simulink model "ADCCalibrationCAN"  (R2026a)
settings: Solver=FixedStepAuto  StopTime=inf  FixedStep=Ts_CPU  EnableMultiTasking=on
InitFcn:
  | Ts = 1e-4;
  | Tcpu = 50e-6; %Controller sample time
  | 
  | % PMSM parameters
  | PM = 0.03; % Permanent magnet flux linkage
  | Ld = 2e-4;  % d-axis inductance
  | Lq = 2e-4;  % q-axis inductance
  | L0 = 2e-4;  % 0-axis inductance
  | Rs = 0.013; % Stator resistance
  | N = 6; % Number of pole pairs
  | J = 0.2; % Moment of inertia
  | 
  | % encoder parameters
  | numSlits = 2000; % number of slits
  | pulseSigOffset = 0; % index pulse signal offset
  | shaftInitPos = 0; % motor shaft initial position
  | 
  | % DAC parameters
  | gain = 0.1;
  | bias = 0;
  | 
  | % circuit parameters
  | Vdc = 48;
  | 
  | % real-time parameters
  | ts_FPGA_clk = 5e-9;
  | ts_FPGA_mdl = 1e-6;
  | 
  | % Real-time processor or embedded controller
  | RTorTTL = 1; % 1: Real-time processor,    0: embedded controller
  | 
  | % sample times
  | f_base = 200e6;
  | PWM_frequency = 20e3;
  | ts_FPGA_clk = 1/f_base;
  | ts_FPGA_mdl =1e-6;
undefined symbols (not defined in the file or in its folder): Foc_Ki_IxTcpu, Foc_Kp_I, IO334, IO334_iDAC_bias, IO334_iDAC_gain, Maxon_645604_J, Maxon_645604_lambda_pm, Maxon_645604_Ld, Maxon_645604_Lq, Maxon_645604_Np, Maxon_645604_Rs, Maxon_645604_StaticF, Maxon_645604_ViscousF, PMSM3P2LInverter_limited, PMSM_3P2L_Inverter_Plant, Ts_CAN_Tx, Ts_CPU, Ts_UI
libraries: speedgoatlib_hdlCoder_IO3xx x31, canmsglib x7, speedgoatlib_IO611 x3, pwm_cpulib x1, quadrature_cpulib x1, resolver_cpulib x1
(part 1 of 2)
settings Model: DataDictionary=PMSM3P2LInverterDd.sldd  EnableAccessToBaseWorkspace=off  SimulationMode=external  ExtModeEnableFloating=off  Creator=chrisz  LastModifiedBy=mathieu.lu-dac
settings SolverCC: ConcurrentTasks=on  PositivePriorityOrder=on
settings OptimizationCC: ConditionallyExecuteInputs=off  OptimizeBlockIOStorage=off
settings DebuggingCC: AlgebraicLoopMsg=error  SingleTaskRateTransMsg=error  TasksWithSamePriorityMsg=none  ParameterOverflowMsg=warning  ParameterUnderflowMsg=warning
settings HardwareCC: ProdBitPerLong=64.0  ProdHWDeviceType=Intel->x86-64 (Linux 64)  TargetBitPerPointer=64.0  TargetBitPerSizeT=64.0  TargetBitPerPtrDiffT=64.0  TargetLongLongMode=on  TargetIntDivRoundTo=Zero  TargetEndianess=LittleEndian  TargetWordSize=64.0  TargetHWDeviceType=Custom Processor->MATLAB Host Computer
settings RTWCC: SystemTargetFile=speedgoat.tlc  TemplateMakefile=slrealtime_default_tmf  Toolchain=Simulink Real-Time Toolchain  BuildConfiguration=Faster Runs  TargetLang=C++  Description=Speedgoat Real-Time Target Machine
settings SimulinkRealTimeTargetCC: SLRTFileLogMaxRuns=1.0  MultiwordLength=2048.0
settings SimscapeCC: SimscapeNominalValues="[{\"value\":\"1\",\"unit\":\"A\"},{\"value\":\"1\",\"unit\":\"bar\"},{\"value\":\"1\",\"unit\":\"cm^2\"},{\"value\":\"1\",\"unit\":\"cm^3/s\"},{\"value\":\"1\",\"unit\":\"kJ/kg\"},{\"value\":\"1\",\"unit\":\"kW\"},{\"value\":\"1\",\"unit\":\"l\"},{\"value\":\"1\",\"unit\":\"N\"},{\"value\":\"1\",\"unit\":\"N*m\"},{\"value\":\"1\",\"unit\":\"V\"}]"  SimscapeLogType=none  SimscapeLogDataHistory=5000.0

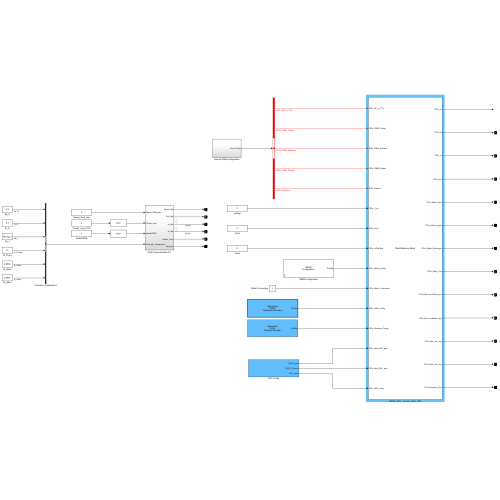
[thumbnail: Simulink's stored preview of the top-level diagram]
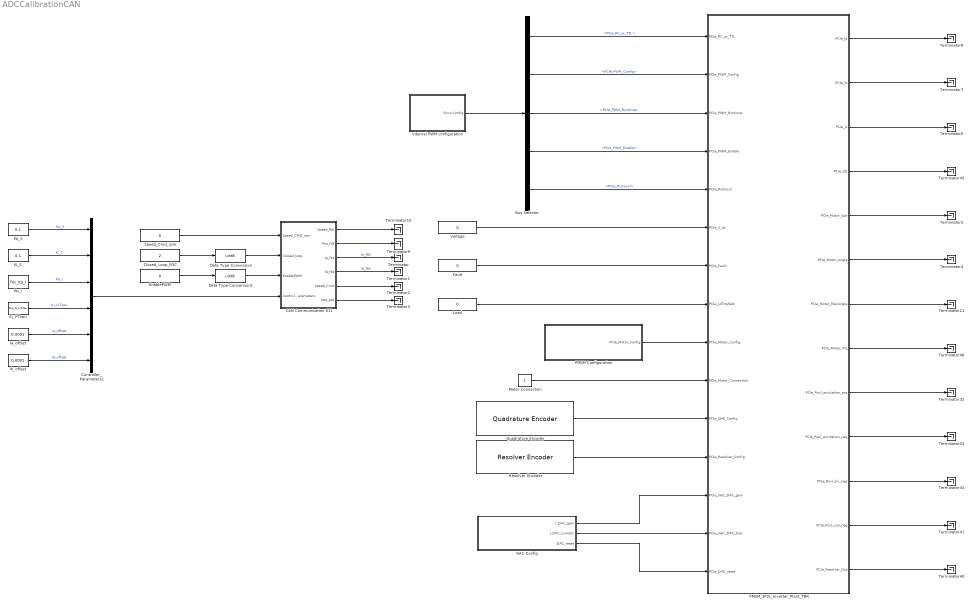
== system ADCCalibrationCAN ==
  Bus Selector : BusSelector  OutputSignals=PCIe_RC_or_TTL,PCIe_PWM_Config,PCIe_PWM_Runtime,PCIe_PWM_Enable,PCIe_Protocol
  CAN Communication 611 : Subsystem
  Closed_Loop_FOC : Constant  Value=2  OutDataTypeStr=uint8  SampleTime=Ts_UI
  Controller_Parameters1 : BusCreator  Inputs=6
  DAC Config : Subsystem
  Data Type Conversion : DataTypeConversion  OutDataTypeStr=uint8  SaturateOnIntegerOverflow=off  RndMeth=Floor
  Data Type Conversion1 : DataTypeConversion  OutDataTypeStr=uint8  SaturateOnIntegerOverflow=off  RndMeth=Floor
  EnablePWM : Constant  Value=0  OutDataTypeStr=boolean  SampleTime=Ts_UI
  Fault : Constant  Value=0  OutDataTypeStr=uint32  SampleTime=Ts_UI
  Ia_offset : Constant  Value=0.0001  OutDataTypeStr=single  SampleTime=Ts_UI
  Ib_offset : Constant  Value=0.0001  OutDataTypeStr=single  SampleTime=Ts_UI
  Internal PWM configuration : Subsystem
  Ki_S : Constant  Value=0.1  OutDataTypeStr=single  SampleTime=Ts_UI
  Ki_i*Tcpu : Constant  Value=Foc_Ki_IxTcpu  OutDataTypeStr=single  SampleTime=Ts_UI
  Kp_I : Constant  Value=Foc_Kp_I  OutDataTypeStr=single  SampleTime=Ts_UI
  Kp_S : Constant  Value=0.1  OutDataTypeStr=single  SampleTime=Ts_UI
  Load : Constant  Value=0  OutDataTypeStr=single  SampleTime=Ts_UI
  Motor Connection : Constant  OutDataTypeStr=boolean
  PMSM Configuration : Subsystem  InitFcn=|  mask(PMSM Configuration){portConfig=Torque, Trq_N_mode=0, Ts=Ts_CPU, Pp=Maxon_645604_Np, Rs=Maxon_645604_Rs, Ld=Maxon_645604_Ld, Lq=Maxon_645604_Lq, lambda_pm=Maxon_645604_lambda_pm, J=Maxon_645604_J, B=Maxon_645604_ViscousF*100, f=Maxon_645604_StaticF}
      | mcb.internal.manageMCBResource('register',gcbh);
      | mcb.internal.logDDUXData;
      mask prompts: portConfig "mcb:PlantLib:CfgMechInCfg"; Ts "mcb:PlantLib:CfgTs"; Pp "mcb:PlantLib:PMSMCfgPp"; Rs "mcb:PlantLib:PMSMCfgRs"; Ld "mcb:PlantLib:PMSMCfgLd"; Lq "mcb:PlantLib:PMSMCfgLq"; lambda_pm "mcb:PlantLib:PMSMCfgLambda"; J "mcb:PlantLib:PMSMCfgJ"; B "mcb:PlantLib:PMSMCfgB"; f "mcb:PlantLib:PMSMCfgf"
      mask help: mcb:PlantLib:PMSMCfgDes
      mask Help: eval('mcb_helpview(''pmsmhdlconfig'')')
      mask TypeOptions portConfig: mcb:PlantLib:CfgTorque | mcb:PlantLib:CfgSpd
      mask Callback portConfig:
      | %Do not run initialization code if model is running
      | invalidStatus = {'external','running','compiled','restarting','paused','terminating'};
      | if ~any(strcmpi(get_param(bdroot(gcb),'SimulationStatus'),invalidStatus))
      |     % Check the value selected in the pop-up
      |     mask = Simulink.Mask.get(gcb);
      |     portConfigStr = get_param(gcb, 'portConfig');
      |     if strcmp(portConfigStr, 'Torque')
      |         % Set Trq_N_mode value to 0
      |         mask.getParameter('Trq_N_mode').Value = '0';
      | 
      |     elseif strcmp(portConfigStr, 'Speed')
      |         % Set Trq_N_mode value to 2
      |         mask.getParameter('Trq_N_mode').Value = '1';
      | 
      |     end
      | end
      mask DialogControl DescGroupVar Prompt: mcb:PlantLib:PMSMCfgTitle
      mask DialogControl ParameterGroupVar Prompt: mcb:PlantLib:CfgBlk
      mask DialogControl portConfig Prompt: Mechanical input configuration:
      mask DialogControl Ts Prompt: Sample time (s):
      mask DialogControl Container4 Prompt: mcb:PlantLib:CfgParam
      mask DialogControl Pp Prompt: Number of pole pairs:
      mask DialogControl Rs Prompt: Stator resistance per phase (Ohm):
      mask DialogControl Ld Prompt: Stator d-axis inductance (H):
      mask DialogControl Lq Prompt: Stator q-axis inductance (H):
      mask DialogControl lambda_pm Prompt: Permanent flux linkage constant (Wb):
      mask DialogControl J Prompt: Inertia (kgm^2):
      mask DialogControl B Prompt: Viscous damping (Nm/rad/s):
      mask DialogControl f Prompt: Static friction (Nm):
      mask Display:
      | disp('PMSM\nConfiguration');
      | port_label('output',1,'Config');
  PMSM_3P2L_Inverter_Plant_TBR : Subsystem
      mask Display: disp('Plant Bitstream Block')
  Quadrature Encoder : quadrature_cpulib/Quadrature Encoder  FPGA_freq=f_FPGA  n_channels=[1]  sel_scaling=FPGA  useSpeed=off  usePosition=on  numOfSlots=Maxon_Mile_Nslits  sigAswitchOn=[180]  sigBswitchOff=[90]  sigBswitchOn=[270]  sigAdismissEn=off  sigAdismissSingle=on  sigAdismissHigh=on  sigBdismissEn=off  sigBdismissSingle=on  sigBdismissHigh=on
      settings: SourceProductName=Quadrature CPU Library
  Resolver Encoder : resolver_cpulib/Resolver Encoder  Ts=Ts_UI  ts_resolver=ts_FPGA_mdl  n_channels=1  sel_scaling=FPGA  useSpeed=on  usePosition=off  pole_pairs=1  gain_dynamic=off  gainVector=[1, 1, 1, 1]  offset_dynamic=off  offsetVector=[0, 0, 0, 0]  exct_freq=2  angle_offset=0  exct_amplitude=10  position_init_enb=off  rotor_position=90  int_exct_enb=off  exct_out_enb=off  phase_delay=0  time_step_delay=0  adcRange=2.5  dacRange=2.5
      settings: SourceProductName=Resolver CPU Library
  Speed_Cmd_rpm : Constant  Value=0  OutDataTypeStr=single  SampleTime=Ts_UI
  Terminator{,1..10,21,32..34,40..41,45..46} (19 alike) : Terminator
  Voltage : Constant  Value=0  OutDataTypeStr=single  SampleTime=Ts_UI
  wires:
  EnablePWM/1 -> Data Type Conversion1/1
  CAN Communication 611/3(Ia_fbk) -> Terminator/1  "Ia_fbk"
  CAN Communication 611/4(Ib_fbk) -> Terminator1/1  "Ib_fbk"
  Controller_Parameters1/1 -> CAN Communication 611/4(Controller_Parameters)
  Speed_Cmd_rpm/1 -> CAN Communication 611/1(Speed_CMD_rpm)
  Closed_Loop_FOC/1 -> Data Type Conversion/1
  Data Type Conversion1/1 -> CAN Communication 611/3(EnablePWM)
  Data Type Conversion/1 -> CAN Communication 611/2(Closed_loop)
  Kp_I/1 -> Controller_Parameters1/3  "Kp_I"
  Ki_i*Tcpu/1 -> Controller_Parameters1/4  "Ki_IxTcpu"
  Ki_S/1 -> Controller_Parameters1/2  "Ki_S"
  Ib_offset/1 -> Controller_Parameters1/6  "Ib_offset"
  Kp_S/1 -> Controller_Parameters1/1  "Kp_S"
  Ia_offset/1 -> Controller_Parameters1/5  "Ia_offset"
  CAN Communication 611/5(Speed_Cmd) -> Terminator2/1
  CAN Communication 611/6(Spd_pot) -> Terminator3/1
  PMSM_3P2L_Inverter_Plant_TBR/1(PCIe_Ia) -> Terminator8/1
  Quadrature Encoder/1 -> PMSM_3P2L_Inverter_Plant_TBR/11(PCIe_QAE_Config)
  PMSM_3P2L_Inverter_Plant_TBR/5(PCIe_Motor_Spd) -> Terminator5/1
  PMSM_3P2L_Inverter_Plant_TBR/2(PCIe_Ib) -> Terminator7/1
  Bus Selector/1 -> PMSM_3P2L_Inverter_Plant_TBR/1(PCIe_RC_or_TTL)  "<PCIe_RC_or_TTL>"
  PMSM_3P2L_Inverter_Plant_TBR/11(PCIe_Rsvl_sin_neg) -> Terminator34/1
  DAC Config/1(I_DAC_gain) -> PMSM_3P2L_Inverter_Plant_TBR/13(PCIe_Iabc_DAC_gain)
  PMSM_3P2L_Inverter_Plant_TBR/10(PCIe_Rsvl_excitation_neg) -> Terminator33/1
  PMSM_3P2L_Inverter_Plant_TBR/7(PCIe_Motor_ElecAngle) -> Terminator21/1
  PMSM_3P2L_Inverter_Plant_TBR/4(PCIe_Idc) -> Terminator45/1
  Bus Selector/5 -> PMSM_3P2L_Inverter_Plant_TBR/5(PCIe_Protocol)  "<PCIe_Protocol>"
  PMSM_3P2L_Inverter_Plant_TBR/3(PCIe_Ic) -> Terminator6/1
  Internal PWM configuration/1(Simu Config) -> Bus Selector/1
  Voltage/1 -> PMSM_3P2L_Inverter_Plant_TBR/6(PCIe_V_dc)
  Fault/1 -> PMSM_3P2L_Inverter_Plant_TBR/7(PCIe_Fault)
  Load/1 -> PMSM_3P2L_Inverter_Plant_TBR/8(PCIe_LdTrq/Spd)
  Resolver Encoder/1 -> PMSM_3P2L_Inverter_Plant_TBR/12(PCIe_Resolver_Config)
  Bus Selector/3 -> PMSM_3P2L_Inverter_Plant_TBR/3(PCIe_PWM_Runtime)  "<PCIe_PWM_Runtime>"
  PMSM_3P2L_Inverter_Plant_TBR/9(PCIe_Rsvl_excitation_pos) -> Terminator32/1
  Bus Selector/4 -> PMSM_3P2L_Inverter_Plant_TBR/4(PCIe_PWM_Enable)  "<PCIe_PWM_Enable>"
  DAC Config/3(DAC_reset) -> PMSM_3P2L_Inverter_Plant_TBR/15(PCIe_DAC_reset)
  Motor Connection/1 -> PMSM_3P2L_Inverter_Plant_TBR/10(PCIe_Motor_Connection)
  PMSM_3P2L_Inverter_Plant_TBR/8(PCIe_Motor_Trq) -> Terminator46/1
  PMSM_3P2L_Inverter_Plant_TBR/13(PCIe_Resolver_Out) -> Terminator40/1
  PMSM_3P2L_Inverter_Plant_TBR/12(PCIe_Rsvl_cos_neg) -> Terminator41/1
  DAC Config/2(I_DAC_Current) -> PMSM_3P2L_Inverter_Plant_TBR/14(PCIe_Iabc_DAC_bias)
  Bus Selector/2 -> PMSM_3P2L_Inverter_Plant_TBR/2(PCIe_PWM_Config)  "<PCIe_PWM_Config>"
  PMSM_3P2L_Inverter_Plant_TBR/6(PCIe_Motor_Angle) -> Terminator4/1
  CAN Communication 611/2(Pos_fdk) -> Terminator9/1
  CAN Communication 611/1(Speed_fbk) -> Terminator10/1
  PMSM Configuration/1(PCIe_Motor_Config) -> PMSM_3P2L_Inverter_Plant_TBR/9(PCIe_Motor_Config)

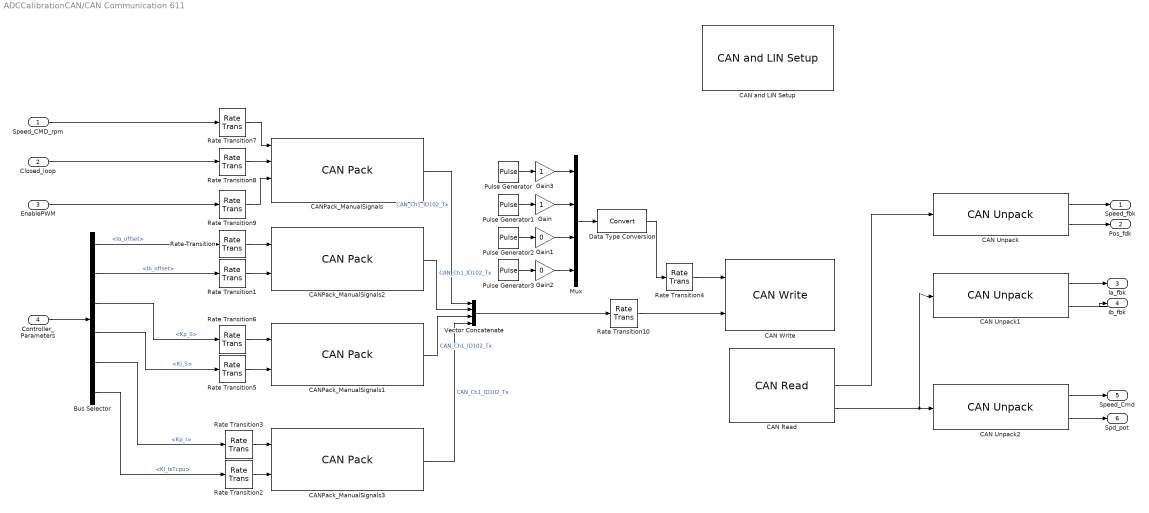
== system ADCCalibrationCAN/CAN Communication 611 ==
  Speed_CMD_rpm : Inport
  Closed_loop : Inport  Port=2
  EnablePWM : Inport  Port=3
  Controller_Parameters : Inport  Port=4
  Bus Selector : BusSelector  OutputSignals=Ia_offset,Ib_offset,Kp_S,Ki_S,Kp_I,Ki_IxTcpu
  "CAN Read " : speedgoatlib_IO611/CAN Read   moduleType=IO611  id=1  channel=1  canType=CAN (HS)  useBusOut=on  HasMulRead=Specify by IDs  MsgIDlist=[1 2]  isEFF=off  LabelInHex=on  enableInput=off  ts=1e-3  initValues=[611 1 0.001 0 1 1 0 1 0 2 2 1 2]
      settings: LibrarySourceBlock=speedgoatlib_CANLIN_OfA2/CAN/CAN Read  SourceProductName=IO611
  CAN Unpack : canmsglib/CAN Unpack  MsgList=(none)  MsgName=Speed_TI_Out  MsgIDType=Standard (11-bit identifier)  MsgIdentifier=1  MsgLength=8  SignalInfo={ 'Speed_fbk', '0', '32', 'LE', 'single', 'Standard', '0', '1', '0', '-Inf', 'Inf'; 'Pos_fbk', '32', '32', 'LE', 'single', 'Standard', '0', '1', '0', '-Inf', 'Inf' }  IDPort=off  TimestampPort=off  ErrorPort=off  RemotePort=off  LengthPort=off  StatusPort=off  ApplyMinMax=off
      settings: LibrarySourceBlock=canlib/CAN Unpack
  CAN Unpack1 : canmsglib/CAN Unpack  MsgList=(none)  MsgName=I_TI_Out  MsgIDType=Standard (11-bit identifier)  MsgIdentifier=2  MsgLength=8  SignalInfo={ 'Ia', '0', '32', 'LE', 'single', 'Standard', '0', '1', '0', '-Inf', 'Inf'; 'Ib', '32', '32', 'LE', 'single', 'Standard', '0', '1', '0', '-Inf', 'Inf' }  IDPort=off  TimestampPort=off  ErrorPort=off  RemotePort=off  LengthPort=off  StatusPort=off  ApplyMinMax=off
      settings: LibrarySourceBlock=canlib/CAN Unpack
  CAN Unpack2 : canmsglib/CAN Unpack  MsgList=(none)  MsgName=Speed_Cmd_fbk  MsgIDType=Standard (11-bit identifier)  MsgIdentifier=2  MsgLength=8  SignalInfo={ 'Speed_Cmd', '0', '32', 'LE', 'single', 'Standard', '0', '1', '0', '-Inf', 'Inf'; 'Spd_pot', '32', '32', 'LE', 'single', 'Standard', '0', '1', '0', '-Inf', 'Inf' }  IDPort=off  TimestampPort=off  ErrorPort=off  RemotePort=off  LengthPort=off  StatusPort=off  ApplyMinMax=off
      settings: LibrarySourceBlock=canlib/CAN Unpack
  "CAN Write " : speedgoatlib_IO611/CAN Write   moduleType=IO611  id=1  channel=1  canType=CAN (HS)  useBusIn=on  numOfMsg=4  enableInput=on  enableStatusPort=off  initValues=[611 1 1 0 1 1 0 4 1 1]  ts=Ts_CAN_Tx*5
      settings: LibrarySourceBlock=speedgoatlib_CANLIN_OfA2/CAN/CAN Write  SourceProductName=IO611
  "CAN and LIN Setup " : speedgoatlib_IO611/CAN and LIN Setup   moduleInitValues="[611    1    1   -1   -1]"  id=1  moduleType=IO611  pciSlot=-1  canChn1=CAN (HS)  canChn2=Disabled  canChn3=Disabled  canChn4=Disabled  linChn1=Disabled  linChn2=Disabled  canInitStructArray=[]  canTermStructArray=[]  canChn1InitValues="[2   2   1  31   8   2   1   5   2]"  arbBdrChn1=1.0 MBaud  arbManBdrChn1=[2,1,31,8]  fdBdrChn1=5.0 MBaud  fdManBdrChn1=[2,1,5,2]  canChn2InitValues="[1  200    1   31    8    2    1    5    2]"  arbBdrChn2=10 kBaud  arbManBdrChn2=[200,1,31,8]  fdBdrChn2=5.0 MBaud  fdManBdrChn2=[2,1,5,2]  canChn3InitValues="[1   2   1  31   8   2   1   5   2]"  arbBdrChn3=1.0 MBaud  arbManBdrChn3=[2,1,31,8]  fdBdrChn3=5.0 MBaud  fdManBdrChn3=[2,1,5,2]  canChn4InitValues="[1   2   1  31   8   2   1   5   2]"  arbBdrChn4=1.0 MBaud  arbManBdrChn4=[2,1,31,8]  fdBdrChn4=5.0 MBaud  fdManBdrChn4=[2,1,5,2]  bdrLIN1=19200  linChn1InitValues="[1  19200]"  bdrLIN2=19200  linChn2InitValues="[1  19200]"
      settings: SourceProductName=IO611
  CANPack_ManualSignals : canmsglib/CAN Pack  MsgList=(none)  MsgName=Speed_Cmd  MsgIDType=Standard (11-bit identifier)  MsgIdentifier=0  CANIDInput=off  MsgLength=8  Remote=off  ApplyMinMax=off  BusOutput=on  SignalInfo={ 'Speed_Cmd', '0', '32', 'LE', 'single', 'Standard', '0', '1', '0', '-Inf', 'Inf'; 'Closed_loop', '32', '8', 'LE', 'unsigned', 'Standard', '0', '1', '0', '-Inf', 'Inf'; 'EnablePWM', '40', '8', 'LE', 'unsigned', 'Standard', '0', '1', '0', '-Inf', 'Inf'; 'Filler', '48', '16', 'LE', 'signed', 'Standard', '0', '1', '0', '-Inf', 'Inf' }
      settings: DataFormat=manually specified signals
  CANPack_ManualSignals1 : canmsglib/CAN Pack  MsgList=(none)  MsgName=Speed_Parameters  MsgIDType=Standard (11-bit identifier)  MsgIdentifier=31  CANIDInput=off  MsgLength=8  Remote=off  ApplyMinMax=off  BusOutput=on  SignalInfo={ 'Kp_S', '0', '32', 'LE', 'single', 'Standard', '0', '1', '0', '-Inf', 'Inf'; 'Ki_S', '32', '32', 'LE', 'single', 'Standard', '0', '1', '0', '-Inf', 'Inf' }
      settings: DataFormat=manually specified signals
  CANPack_ManualSignals2 : canmsglib/CAN Pack  MsgList=(none)  MsgName=I_Offsets  MsgIDType=Standard (11-bit identifier)  MsgIdentifier=30  CANIDInput=off  MsgLength=8  Remote=off  ApplyMinMax=off  BusOutput=on  SignalInfo={ 'Ia_offset', '0', '32', 'LE', 'single', 'Standard', '0', '1', '0', '-Inf', 'Inf'; 'Ib_offset', '32', '32', 'LE', 'single', 'Standard', '0', '1', '0', '-Inf', 'Inf' }
      settings: DataFormat=manually specified signals
  CANPack_ManualSignals3 : canmsglib/CAN Pack  MsgList=(none)  MsgName=I_Parameters  MsgIDType=Standard (11-bit identifier)  MsgIdentifier=29  CANIDInput=off  MsgLength=8  Remote=off  ApplyMinMax=off  BusOutput=on  SignalInfo={ 'Kp_I', '0', '32', 'LE', 'single', 'Standard', '0', '1', '0', '-Inf', 'Inf'; 'Ki_I', '32', '32', 'LE', 'single', 'Standard', '0', '1', '0', '-Inf', 'Inf' }
      settings: DataFormat=manually specified signals
  Data Type Conversion : DataTypeConversion  SaturateOnIntegerOverflow=off  RndMeth=Floor
  Gain : Gain
  Gain1 : Gain  Gain=0
  Gain2 : Gain  Gain=0
  Gain3 : Gain
  Mux : Mux
  Pulse Generator : DiscretePulseGenerator  Period=40  PulseWidth=10  SampleTime=Ts_CAN_Tx/10
  Pulse Generator1 : DiscretePulseGenerator  Period=40  PulseWidth=10  PhaseDelay=10  SampleTime=Ts_CAN_Tx/10
  Pulse Generator2 : DiscretePulseGenerator  Period=40  PulseWidth=10  PhaseDelay=20  SampleTime=Ts_CAN_Tx/10
  Pulse Generator3 : DiscretePulseGenerator  Period=40  PulseWidth=10  PhaseDelay=30  SampleTime=Ts_CAN_Tx/10
  Rate Transition{,1..3,5..9} (9 alike) : RateTransition  Integrity=off  Deterministic=off  OutPortSampleTime=Ts_CAN_Tx
  Rate Transition10 : RateTransition  Integrity=off  OutPortSampleTime=Ts_CAN_Tx*5
  Rate Transition4 : RateTransition  Integrity=off  OutPortSampleTime=Ts_CAN_Tx*5
  Vector Concatenate : Concatenate  NumInputs=4
  Speed_fbk : Outport
  Pos_fdk : Outport  Port=2
  Ia_fbk : Outport  Port=3
  Ib_fbk : Outport  Port=4
  Speed_Cmd : Outport  Port=5
  Spd_pot : Outport  Port=6
  wires:
  "CAN Read "/2 -> CAN Unpack/1
  CAN Unpack/1 -> Speed_fbk/1
  CAN Unpack/2 -> Pos_fdk/1
  CAN Unpack1/1 -> Ia_fbk/1
  "CAN Read "/3 -> CAN Unpack1/1, CAN Unpack2/1
  CAN Unpack1/2 -> Ib_fbk/1
  CAN Unpack2/2 -> Spd_pot/1
  CAN Unpack2/1 -> Speed_Cmd/1
  Bus Selector/3 -> Rate Transition6/1  "<Kp_S>"
  Bus Selector/4 -> Rate Transition5/1  "<Ki_S>"
  Bus Selector/2 -> Rate Transition1/1  "<Ib_offset>"
  Bus Selector/1 -> Rate Transition/1  "<Ia_offset>"
  Controller_Parameters/1 -> Bus Selector/1
  Bus Selector/6 -> Rate Transition2/1  "<Ki_IxTcpu>"
  Bus Selector/5 -> Rate Transition3/1  "<Kp_I>"
  CANPack_ManualSignals1/1 -> Vector Concatenate/3  "CAN_Ch1_ID102_Tx"
  CANPack_ManualSignals2/1 -> Vector Concatenate/2  "CAN_Ch1_ID102_Tx"
  Pulse Generator/1 -> Gain3/1
  CANPack_ManualSignals/1 -> Vector Concatenate/1  "CAN_Ch1_ID102_Tx"
  Data Type Conversion/1 -> Rate Transition4/1
  Pulse Generator2/1 -> Gain1/1
  Pulse Generator1/1 -> Gain/1
  Mux/1 -> Data Type Conversion/1
  CANPack_ManualSignals3/1 -> Vector Concatenate/4  "CAN_Ch1_ID102_Tx"
  Pulse Generator3/1 -> Gain2/1
  Rate Transition/1 -> CANPack_ManualSignals2/1
  Rate Transition1/1 -> CANPack_ManualSignals2/2
  Rate Transition6/1 -> CANPack_ManualSignals1/1
  Rate Transition5/1 -> CANPack_ManualSignals1/2
  Rate Transition3/1 -> CANPack_ManualSignals3/1
  Rate Transition2/1 -> CANPack_ManualSignals3/2
  Speed_CMD_rpm/1 -> Rate Transition7/1
  Rate Transition7/1 -> CANPack_ManualSignals/1
  Closed_loop/1 -> Rate Transition8/1
  Rate Transition8/1 -> CANPack_ManualSignals/2
  EnablePWM/1 -> Rate Transition9/1
  Rate Transition9/1 -> CANPack_ManualSignals/3
  Gain3/1 -> Mux/1
  Gain/1 -> Mux/2
  Gain1/1 -> Mux/3
  Gain2/1 -> Mux/4
  Vector Concatenate/1 -> Rate Transition10/1
  Rate Transition4/1 -> "CAN Write "/1
  Rate Transition10/1 -> "CAN Write "/2

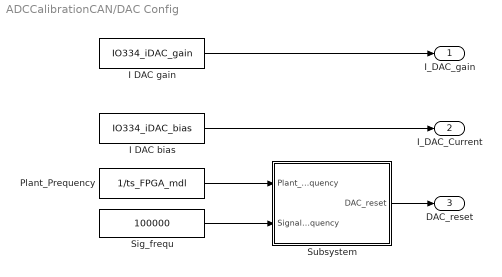
== system ADCCalibrationCAN/DAC Config ==
  I DAC bias : Constant  Value=IO334_iDAC_bias  OutDataTypeStr=single  SampleTime=Ts_UI
  I DAC gain : Constant  Value=IO334_iDAC_gain  OutDataTypeStr=single  SampleTime=Ts_UI
  Plant_Prequency : Constant  Value=1/ts_FPGA_mdl  SampleTime=Ts_UI
  Sig_frequ : Constant  Value=100000  VectorParams1D=off  SampleTime=Ts_UI
  Subsystem : Subsystem
  I_DAC_gain : Outport
  I_DAC_Current : Outport  Port=2
  DAC_reset : Outport  Port=3
  wires:
  Subsystem/1(DAC_reset) -> DAC_reset/1
  Plant_Prequency/1 -> Subsystem/1(Plant_frequency)
  Sig_frequ/1 -> Subsystem/2(SignalFrequency)
  I DAC gain/1 -> I_DAC_gain/1
  I DAC bias/1 -> I_DAC_Current/1

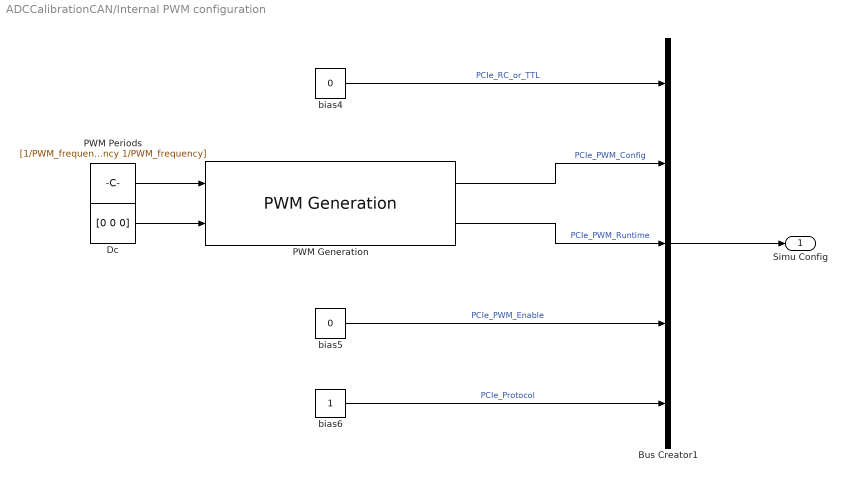
== system ADCCalibrationCAN/Internal PWM configuration ==
  Bus Creator1 : BusCreator  Inputs=5
  Dc : Constant  Value=[0 0 0]  OutDataTypeStr=double
  PWM Generation : pwm_cpulib/PWM Generation  f_FPGA=f_FPGA  n_channels=3  sel_scaling=CPU  protection_param=Disabled: A and B can be high at the same moment  deadband_sec=0  natural_update=At period starts  delay=0  trigger_duration_sec=[1e-6]  trigger_period_start=off  trigger_half_of_the_period=off  trigger_a_on=off  trigger_a_off=off  trigger_b_on=off  trigger_b_off=off  bit_width_pwm_gen=24  invert_a=off  invert_b=off  invert_c=off  showPhaseInput=off
      settings: SourceProductName=PWM CPU Library
  PWM Periods : Constant  Value=[1/PWM_frequency 1/PWM_frequency 1/PWM_frequency]  OutDataTypeStr=double
  bias4 : Constant  Value=0  OutDataTypeStr=boolean  SampleTime=Ts_UI
  bias5 : Constant  Value=0  OutDataTypeStr=boolean  SampleTime=Ts_UI
  bias6 : Constant  OutDataTypeStr=boolean  SampleTime=Ts_UI
  Simu Config : Outport
  wires:
  PWM Generation/2 -> Bus Creator1/3  "PCIe_PWM_Runtime"
  bias6/1 -> Bus Creator1/5  "PCIe_Protocol"
  PWM Generation/1 -> Bus Creator1/2  "PCIe_PWM_Config"
  Bus Creator1/1 -> Simu Config/1
  bias4/1 -> Bus Creator1/1  "PCIe_RC_or_TTL"
  bias5/1 -> Bus Creator1/4  "PCIe_PWM_Enable"
  PWM Periods/1 -> PWM Generation/1
  Dc/1 -> PWM Generation/2

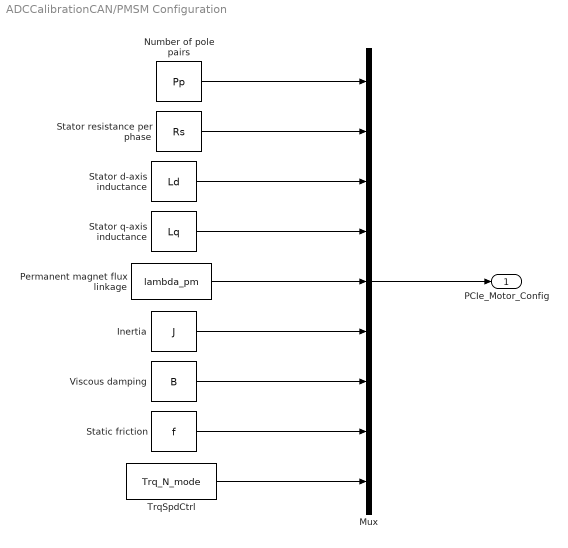
== system ADCCalibrationCAN/PMSM Configuration ==
  Inertia : Constant  Value=J  OutDataTypeStr=single  SampleTime=Ts
  Mux : Mux  Inputs=9
  Number of pole pairs : Constant  Value=Pp  OutDataTypeStr=single  SampleTime=Ts
  Permanent magnet flux linkage : Constant  Value=lambda_pm  OutDataTypeStr=single  SampleTime=Ts
  Static friction : Constant  Value=f  OutDataTypeStr=single  SampleTime=Ts
  Stator d-axis inductance : Constant  Value=Ld  OutDataTypeStr=single  SampleTime=Ts
  Stator q-axis inductance : Constant  Value=Lq  OutDataTypeStr=single  SampleTime=Ts
  Stator resistance per phase : Constant  Value=Rs  OutDataTypeStr=single  SampleTime=Ts
  TrqSpdCtrl : Constant  Value=Trq_N_mode  OutDataTypeStr=single  SampleTime=Ts
  Viscous damping : Constant  Value=B  OutDataTypeStr=single  SampleTime=Ts
  PCIe_Motor_Config : Outport
  wires:
  Permanent magnet flux linkage/1 -> Mux/5
  Stator resistance per phase/1 -> Mux/2
  TrqSpdCtrl/1 -> Mux/9
  Static friction/1 -> Mux/8
  Viscous damping/1 -> Mux/7
  Mux/1 -> PCIe_Motor_Config/1
  Inertia/1 -> Mux/6
  Stator q-axis inductance/1 -> Mux/4
  Stator d-axis inductance/1 -> Mux/3
  Number of pole pairs/1 -> Mux/1

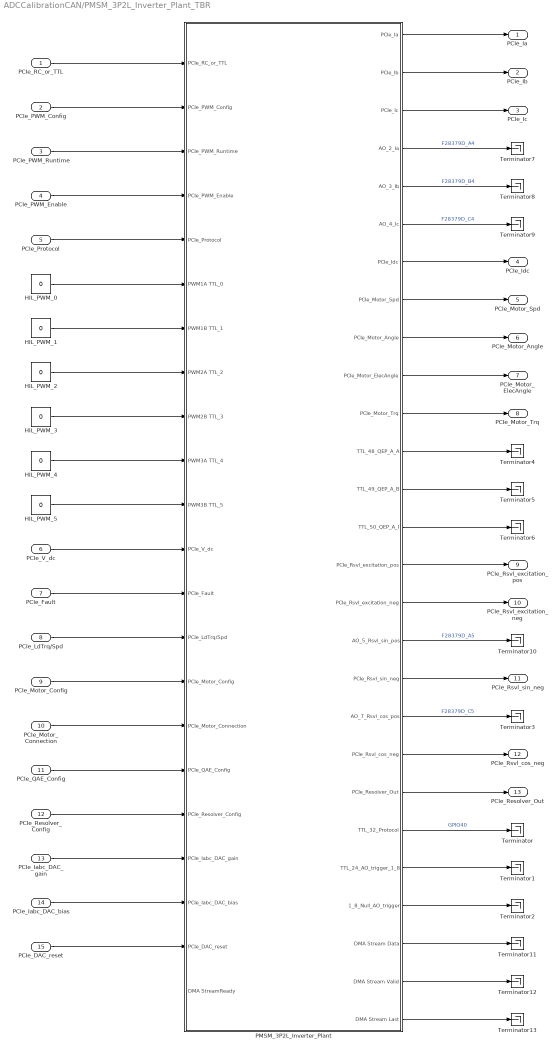
== system ADCCalibrationCAN/PMSM_3P2L_Inverter_Plant_TBR ==
  PCIe_RC_or_TTL : Inport
  PCIe_PWM_Config : Inport  Port=2
  PCIe_PWM_Runtime : Inport  Port=3
  PCIe_PWM_Enable : Inport  Port=4
  PCIe_Protocol : Inport  Port=5
  PCIe_V_dc : Inport  Port=6
  PCIe_Fault : Inport  Port=7
  PCIe_LdTrq/Spd : Inport  Port=8
  PCIe_Motor_Config : Inport  Port=9
  PCIe_Motor_Connection : Inport  Port=10
  PCIe_QAE_Config : Inport  Port=11
  PCIe_Resolver_Config : Inport  Port=12
  PCIe_Iabc_DAC_gain : Inport  Port=13
  PCIe_Iabc_DAC_bias : Inport  Port=14
  PCIe_DAC_reset : Inport  Port=15
  HIL_PWM_{0..5} (6 alike) : Constant  Value=0  OutDataTypeStr=boolean
  PMSM_3P2L_Inverter_Plant : Subsystem  mask(Speedgoat IO334-325k Interface Block){module_id=1, slot=-1, ts=-1, dacGain_1=+/- 10.0V, dacActiv_1=off, dacGain_2=+/- 2.5V, dacActiv_2=on, dacGain_3=+/- 2.5V, dacActiv_3=on, dacGain_4=+/- 2.5V, dacActiv_4=on, dacGain_5=+/- 2.5V, dacActiv_5=on, dacGain_6=+/- 10.0V, dacActiv_6=off, dacGain_7=+/- 2.5V, dacActiv_7=on, dacGain_8=+/- 10.0V, dacActiv_8=off, dacGain_9=+/- 10.0V, dacActiv_9=off, dacGain_10=+/- 10.0V, dacActiv_10=off, dacGain_11=+/- 10.0V, dacActiv_11=off, dacGain_12=+/- 10.0V, dacActiv_12=off, dacGain_13=+/- 10.0V, dacActiv_13=off, dacGain_14=+/- 10.0V, dacActiv_14=off, dacGain_15=+/- 10.0V, dacActiv_15=off, dacGain_16=+/- 10.0V, dacActiv_16=off, PullRPort0=pull-up 3.3V, VioPort0=3.3V, PullRPort1=pull-up 3.3V, VioPort1=3.3V, PullRPort2=pull-up 3.3V, VioPort2=3.3V, PullRPort3=pull-up 3.3V, VioPort3=3.3V, PullRPort4=pull-up 3.3V, VioPort4=3.3V, PullRPort5=pull-up 3.3V, VioPort5=3.3V, PullRPort6=pull-up 3.3V, VioPort6=3.3V, fpga_sync_mode=on, reset_mode=on, reset_mode_stop=on, FpgaFreq=200}
      mask prompts: module_id "FPGA Module Identifier:"; slot "PCI slot (-1: autosearch):"; ts "Sample time:"; dacGain_1 "DAC Ch 01 Range"; dacActiv_1 "Active"; dacGain_2 "DAC Ch 02 Range"; dacActiv_2 "Active"; dacGain_3 "DAC Ch 03 Range"; dacActiv_3 "Active"; dacGain_4 "DAC Ch 04 Range"; dacActiv_4 "Active"; dacGain_5 "DAC Ch 05 Range"; dacActiv_5 "Active"; dacGain_6 "DAC Ch 06 Range"; dacActiv_6 "Active"; dacGain_7 "DAC Ch 07 Range"; dacActiv_7 "Active"; dacGain_8 "DAC Ch 08 Range"; dacActiv_8 "Active"; dacGain_9 "DAC Ch 09 Range"; dacActiv_9 "Active"; dacGain_10 "DAC Ch 10 Range"; dacActiv_10 "Active"; dacGain_11 "DAC Ch 11 Range"; dacActiv_11 "Active"; dacGain_12 "DAC Ch 12 Range"; dacActiv_12 "Active"; dacGain_13 "DAC Ch 13 Range"; dacActiv_13 "Active"; dacGain_14 "DAC Ch 14 Range"; dacActiv_14 "Active"; dacGain_15 "DAC Ch 15 Range"; dacActiv_15 "Active"; dacGain_16 "DAC Ch 16 Range"; dacActiv_16 "Active"; PullRPort0 "pull resistor"; VioPort0 "I/O voltage"; PullRPort1 "pull resistor"; VioPort1 "I/O voltage"; PullRPort2 "pull resistor"; VioPort2 "I/O voltage"; PullRPort3 "pull resistor"; VioPort3 "I/O voltage"; PullRPort4 "pull resistor"; VioPort4 "I/O voltage"; PullRPort5 "pull resistor"; VioPort5 "I/O voltage"; PullRPort6 "pull resistor"; VioPort6 "I/O voltage"; fpga_sync_mode "Run FPGA only when target application runs"; reset_mode "Reset FPGA states on start"; reset_mode_stop "Reset FPGA states on stop"; FpgaFreq "FPGA Frequency [MHz]"
      mask help: Simulink Real-Time Interface Block for Speedgoat IO334-325k.
      mask init:
      | hdlslrt.backend.mfpgaparameters;
      | if sg.hdlc.utils.compareMatlabVersion('~=', 'R2025a')
      | 	sg.hdlc.warning(['The interface model that you are attempting to use was generated ',...
      | 		'in MATLAB R2025a and may not be compatible with the version you are currently using. ',...
      | 		'Attempting to use this interface model in a different MATLAB release can lead to ',...
      | 		'application crashes or other unpredictable behavior. ',...
      | 		'In order to avoid this and ensure stability and correct functionality, ',...
      | 		'we highly recommend regenerating the model with your current MATLAB release.']);
      | end
      mask Help: eval('sg.hdlc.utils.help.show(''refentry_workflow_generated_model'',''isHdlcHelp'', true)')
      mask TypeOptions dacGain_1: AD5547 Setup/dacGain_1
      mask TypeOptions dacActiv_1: AD5547 Setup/dacActiv_1
      mask TypeOptions dacGain_2: AD5547 Setup/dacGain_2
      mask TypeOptions dacActiv_2: AD5547 Setup/dacActiv_2
      mask TypeOptions dacGain_3: AD5547 Setup/dacGain_3
      mask TypeOptions dacActiv_3: AD5547 Setup/dacActiv_3
      mask TypeOptions dacGain_4: AD5547 Setup/dacGain_4
      mask TypeOptions dacActiv_4: AD5547 Setup/dacActiv_4
      mask TypeOptions dacGain_5: AD5547 Setup/dacGain_5
      mask TypeOptions dacActiv_5: AD5547 Setup/dacActiv_5
      mask TypeOptions dacGain_6: AD5547 Setup/dacGain_6
      mask TypeOptions dacActiv_6: AD5547 Setup/dacActiv_6
      mask TypeOptions dacGain_7: AD5547 Setup/dacGain_7
      mask TypeOptions dacActiv_7: AD5547 Setup/dacActiv_7
      mask TypeOptions dacGain_8: AD5547 Setup/dacGain_8
      mask TypeOptions dacActiv_8: AD5547 Setup/dacActiv_8
      mask TypeOptions dacGain_9: AD5547 Setup/dacGain_9
      mask TypeOptions dacActiv_9: AD5547 Setup/dacActiv_9
      mask TypeOptions dacGain_10: AD5547 Setup/dacGain_10
      mask TypeOptions dacActiv_10: AD5547 Setup/dacActiv_10
      mask TypeOptions dacGain_11: AD5547 Setup/dacGain_11
      mask TypeOptions dacActiv_11: AD5547 Setup/dacActiv_11
      mask TypeOptions dacGain_12: AD5547 Setup/dacGain_12
      mask TypeOptions dacActiv_12: AD5547 Setup/dacActiv_12
      mask TypeOptions dacGain_13: AD5547 Setup/dacGain_13
      mask TypeOptions dacActiv_13: AD5547 Setup/dacActiv_13
      mask TypeOptions dacGain_14: AD5547 Setup/dacGain_14
      mask TypeOptions dacActiv_14: AD5547 Setup/dacActiv_14
      mask TypeOptions dacGain_15: AD5547 Setup/dacGain_15
      mask TypeOptions dacActiv_15: AD5547 Setup/dacActiv_15
      mask TypeOptions dacGain_16: AD5547 Setup/dacGain_16
      mask TypeOptions dacActiv_16: AD5547 Setup/dacActiv_16
      mask TypeOptions PullRPort0: Port Settings -2x 0x00590000/PullRPort0
      mask Callback PullRPort0: sg_fpga_HDLCoder_io3xx_2x_m(2);
      mask TypeOptions VioPort0: Port Settings -2x 0x00590000/VioPort0
      mask Callback VioPort0: sg_fpga_HDLCoder_io3xx_2x_m(2);
      mask TypeOptions PullRPort1: Port Settings -2x 0x00590000/PullRPort1
      mask Callback PullRPort1: sg_fpga_HDLCoder_io3xx_2x_m(2);
      mask TypeOptions VioPort1: Port Settings -2x 0x00590000/VioPort1
      mask Callback VioPort1: sg_fpga_HDLCoder_io3xx_2x_m(2);
      mask TypeOptions PullRPort2: Port Settings -2x 0x00590000/PullRPort2
      mask Callback PullRPort2: sg_fpga_HDLCoder_io3xx_2x_m(2);
      mask TypeOptions VioPort2: Port Settings -2x 0x00590000/VioPort2
      mask Callback VioPort2: sg_fpga_HDLCoder_io3xx_2x_m(2);
      mask TypeOptions PullRPort3: Port Settings -2x 0x00590000/PullRPort3
      mask Callback PullRPort3: sg_fpga_HDLCoder_io3xx_2x_m(2);
      mask TypeOptions VioPort3: Port Settings -2x 0x00590000/VioPort3
      mask Callback VioPort3: sg_fpga_HDLCoder_io3xx_2x_m(2);
      mask TypeOptions PullRPort4: Port Settings -2x 0x00590000/PullRPort4
      mask Callback PullRPort4: sg_fpga_HDLCoder_io3xx_2x_m(2);
      mask TypeOptions VioPort4: Port Settings -2x 0x00590000/VioPort4
      mask Callback VioPort4: sg_fpga_HDLCoder_io3xx_2x_m(2);
      mask TypeOptions PullRPort5: Port Settings -2x 0x00590000/PullRPort5
      mask Callback PullRPort5: sg_fpga_HDLCoder_io3xx_2x_m(2);
      mask TypeOptions VioPort5: Port Settings -2x 0x00590000/VioPort5
      mask Callback VioPort5: sg_fpga_HDLCoder_io3xx_2x_m(2);
      mask TypeOptions PullRPort6: Port Settings -2x 0x00590000/PullRPort6
      mask Callback PullRPort6: sg_fpga_HDLCoder_io3xx_2x_m(2);
      mask TypeOptions VioPort6: Port Settings -2x 0x00590000/VioPort6
      mask Callback VioPort6: sg_fpga_HDLCoder_io3xx_2x_m(2);
      mask TypeOptions fpga_sync_mode: IO3xx Setup/fpga_sync_mode
      mask TypeOptions reset_mode: IO3xx Setup/reset_mode
      mask TypeOptions reset_mode_stop: IO3xx Setup/reset_mode_stop
      mask DialogControl DAC Prompt: DAC
      mask DialogControl dacGrp_1 Prompt: Ch 01 to 08
      mask DialogControl dacGrp_2 Prompt: Ch 09 to 16
      mask DialogControl IO33421 Prompt: IO334-21
      mask DialogControl port1 Prompt: Port 1
      mask DialogControl port2 Prompt: Port 2
      mask DialogControl port3 Prompt: Port 3
      mask DialogControl port4 Prompt: Port 4
      mask DialogControl port5 Prompt: Port 5
      mask DialogControl port6 Prompt: Port 6
      mask DialogControl port7 Prompt: Port 7
      mask Display:
      | SetupBlkPath = sghdlc.model.findSystem(gcb, 'LookUnderMasks', 'all', 'FollowLinks', 'on', 'regexp', 'on', 'Name', 'IO3(\d|x){2}\s+Setup' );
      | SetupBlkPath = SetupBlkPath{1};
      | TS = get_param(SetupBlkPath,'timestamp_mcs');
      | disp(sprintf('Speedgoat IO334-325k\n\nTimestamp\n%s\n\nReference Design\nVersion 1.0\n\nMATLAB R2025a\n\nPCIe Link Width: X4\nTiming Severity: error\nRear Plugin: -21\nAurora Mode: None\nAurora Crc: true\nAurora Byteswap: true\nVerifier: off\nVerifier: JTAG\n', TS))
  Terminator{,1..13} (14 alike) : Terminator
  PCIe_Ia : Outport
  PCIe_Ib : Outport  Port=2
  PCIe_Ic : Outport  Port=3
  PCIe_Idc : Outport  Port=4
  PCIe_Motor_Spd : Outport  Port=5
  PCIe_Motor_Angle : Outport  Port=6
  PCIe_Motor_ElecAngle : Outport  Port=7
  PCIe_Motor_Trq : Outport  Port=8
  PCIe_Rsvl_excitation_pos : Outport  Port=9
  PCIe_Rsvl_excitation_neg : Outport  Port=10
  PCIe_Rsvl_sin_neg : Outport  Port=11
  PCIe_Rsvl_cos_neg : Outport  Port=12
  PCIe_Resolver_Out : Outport  Port=13
  wires:
  PMSM_3P2L_Inverter_Plant/1(PCIe_Ia) -> PCIe_Ia/1
  PMSM_3P2L_Inverter_Plant/3(PCIe_Ic) -> PCIe_Ic/1
  PMSM_3P2L_Inverter_Plant/2(PCIe_Ib) -> PCIe_Ib/1
  PMSM_3P2L_Inverter_Plant/7(PCIe_Idc) -> PCIe_Idc/1
  PMSM_3P2L_Inverter_Plant/8(PCIe_Motor_Spd) -> PCIe_Motor_Spd/1
  PMSM_3P2L_Inverter_Plant/9(PCIe_Motor_Angle) -> PCIe_Motor_Angle/1
  PMSM_3P2L_Inverter_Plant/10(PCIe_Motor_ElecAngle) -> PCIe_Motor_ElecAngle/1
  PMSM_3P2L_Inverter_Plant/11(PCIe_Motor_Trq) -> PCIe_Motor_Trq/1
  PMSM_3P2L_Inverter_Plant/15(PCIe_Rsvl_excitation_pos) -> PCIe_Rsvl_excitation_pos/1
  PMSM_3P2L_Inverter_Plant/16(PCIe_Rsvl_excitation_neg) -> PCIe_Rsvl_excitation_neg/1
  PMSM_3P2L_Inverter_Plant/17(AO_5_Rsvl_sin_pos) -> Terminator10/1  "F28379D_A5"
  PMSM_3P2L_Inverter_Plant/18(PCIe_Rsvl_sin_neg) -> PCIe_Rsvl_sin_neg/1
  PMSM_3P2L_Inverter_Plant/20(PCIe_Rsvl_cos_neg) -> PCIe_Rsvl_cos_neg/1
  PMSM_3P2L_Inverter_Plant/21(PCIe_Resolver_Out) -> PCIe_Resolver_Out/1
  PMSM_3P2L_Inverter_Plant/22(TTL_32_Protocol) -> Terminator/1  "GPIO40"
  PMSM_3P2L_Inverter_Plant/23(TTL_24_AO_trigger_1_8) -> Terminator1/1
  PMSM_3P2L_Inverter_Plant/24(1_8_Null_AO_trigger) -> Terminator2/1
  PMSM_3P2L_Inverter_Plant/19(AO_7_Rsvl_cos_pos) -> Terminator3/1  "F28379D_C5"
  PMSM_3P2L_Inverter_Plant/14("TTL_50_QEP_A_I   ") -> Terminator6/1
  PMSM_3P2L_Inverter_Plant/12(TTL_48_QEP_A_A) -> Terminator4/1
  PMSM_3P2L_Inverter_Plant/13(TTL_49_QEP_A_B) -> Terminator5/1
  PMSM_3P2L_Inverter_Plant/6(AO_4_Ic) -> Terminator9/1  "F28379D_C4"
  PMSM_3P2L_Inverter_Plant/4(AO_2_Ia) -> Terminator7/1  "F28379D_A4"
  PMSM_3P2L_Inverter_Plant/5(AO_3_Ib) -> Terminator8/1  "F28379D_B4"
  HIL_PWM_0/1 -> PMSM_3P2L_Inverter_Plant/6(PWM1A TTL_0)
  PCIe_RC_or_TTL/1 -> PMSM_3P2L_Inverter_Plant/1(PCIe_RC_or_TTL)
  PCIe_PWM_Config/1 -> PMSM_3P2L_Inverter_Plant/2(PCIe_PWM_Config)
  PCIe_PWM_Runtime/1 -> PMSM_3P2L_Inverter_Plant/3(PCIe_PWM_Runtime)
  PCIe_PWM_Enable/1 -> PMSM_3P2L_Inverter_Plant/4(PCIe_PWM_Enable)
  PCIe_Protocol/1 -> PMSM_3P2L_Inverter_Plant/5(PCIe_Protocol)
  HIL_PWM_1/1 -> PMSM_3P2L_Inverter_Plant/7(PWM1B TTL_1)
  HIL_PWM_2/1 -> PMSM_3P2L_Inverter_Plant/8(PWM2A TTL_2)
  HIL_PWM_3/1 -> PMSM_3P2L_Inverter_Plant/9(PWM2B TTL_3)
  HIL_PWM_4/1 -> PMSM_3P2L_Inverter_Plant/10(PWM3A TTL_4)
  HIL_PWM_5/1 -> PMSM_3P2L_Inverter_Plant/11(PWM3B TTL_5)
  PCIe_V_dc/1 -> PMSM_3P2L_Inverter_Plant/12(PCIe_V_dc)
  PCIe_Fault/1 -> PMSM_3P2L_Inverter_Plant/13(PCIe_Fault)
  PCIe_LdTrq/Spd/1 -> PMSM_3P2L_Inverter_Plant/14(PCIe_LdTrq/Spd)
  PCIe_Motor_Config/1 -> PMSM_3P2L_Inverter_Plant/15(PCIe_Motor_Config)
  PCIe_Motor_Connection/1 -> PMSM_3P2L_Inverter_Plant/16(PCIe_Motor_Connection)
  PCIe_QAE_Config/1 -> PMSM_3P2L_Inverter_Plant/17(PCIe_QAE_Config)
  PCIe_Resolver_Config/1 -> PMSM_3P2L_Inverter_Plant/18(PCIe_Resolver_Config)
  PCIe_Iabc_DAC_gain/1 -> PMSM_3P2L_Inverter_Plant/19(PCIe_Iabc_DAC_gain)
  PCIe_Iabc_DAC_bias/1 -> PMSM_3P2L_Inverter_Plant/20(PCIe_Iabc_DAC_bias)
  PCIe_DAC_reset/1 -> PMSM_3P2L_Inverter_Plant/21(PCIe_DAC_reset)
  PMSM_3P2L_Inverter_Plant/26(DMA Stream Valid) -> Terminator12/1
  PMSM_3P2L_Inverter_Plant/25(DMA Stream Data) -> Terminator11/1
  PMSM_3P2L_Inverter_Plant/27(DMA Stream Last) -> Terminator13/1

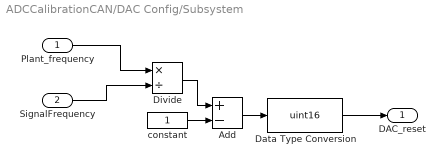
== system ADCCalibrationCAN/DAC Config/Subsystem ==
  Plant_frequency : Inport
  SignalFrequency : Inport  Port=2
  Add : Sum  Inputs=+-
  Data Type Conversion : DataTypeConversion  OutDataTypeStr=uint16  SaturateOnIntegerOverflow=off  RndMeth=Floor
  Divide : Product  Inputs=*/
  constant : Constant  VectorParams1D=off  SampleTime=-1
  DAC_reset : Outport
  wires:
  SignalFrequency/1 -> Divide/2
  Add/1 -> Data Type Conversion/1
  Divide/1 -> Add/1
  Data Type Conversion/1 -> DAC_reset/1
  constant/1 -> Add/2
  Plant_frequency/1 -> Divide/1
